simulink library "xbsEDKLib"  (Simulink 6.1)
libraries: xbsIndex_r4 x58
settings Model: LastModifiedBy=sps

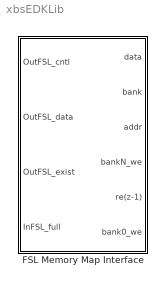
== system xbsEDKLib ==
  FSL Memory Map Interface : Subsystem
      settings: CopyFcn=set_param(gcbh,'LinkStatus','none');
      mask Display:
      | fprintf('','COMMENT: begin icon graphics {110:209:XBlock}');
      | patch([0 110 110 0 ],[0 0 209 209 ],[0.77 0.82 0.91]);
      | patch([25 7 33 7 25 54 62 70 101 76 53 36 61 36 53 76 101 70 62 54 25 ],[61 79 105 131 149 149 141 149 149 124 147 130 105 80 63 86 61 61 69 61 61 ],[.98 .96 .92]);
      | plot([0 0 110 110 0 ],[0 209 209 0 0 ]);
      | fprintf('','COMMENT: end icon graphics');
      | port_label('input',1,'OutFSL_cntl');
      | port_label('input',2,'OutFSL_data');
      | port_label('input',3,'OutFSL_exist');
      | port_label('input',4,'InFSL_full');
      | 
      | port_label('output',1,'data');
      | port_label('output',2,'bank');
      | port_label('output',3,'addr');
      | port_label('output',4,'bankN_we');
      | port_label('output',5,'re(z-1)');
      | port_label('output',6,'bank0_we');

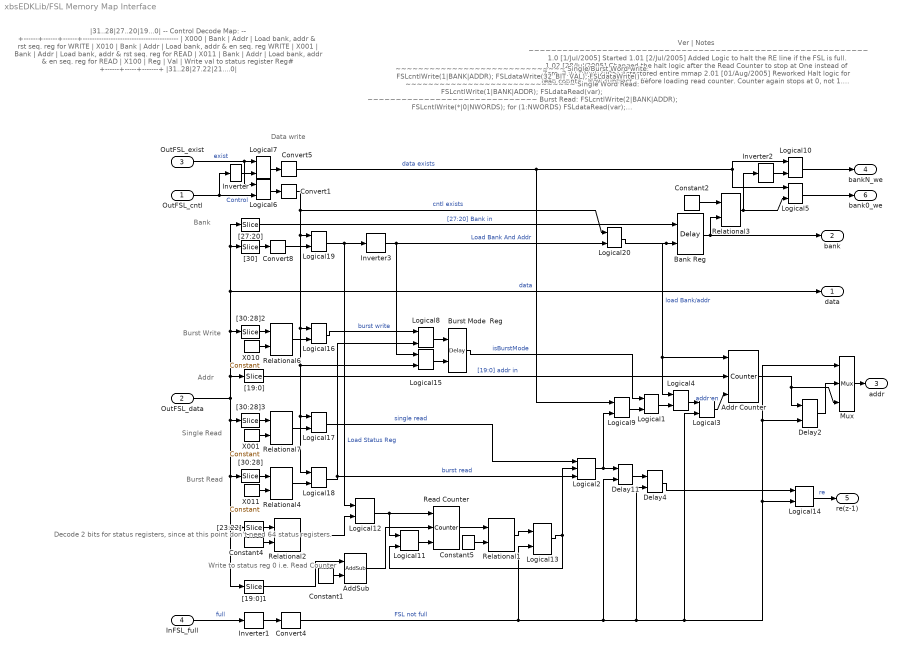
== system xbsEDKLib/FSL Memory Map Interface ==
  note: Ver | Notes
      | ~~~~~~~~~~~~~~~~~~~~~~~~~~~~~~~~~~~~~~~~~~~~~~~~~~~~~~~~~~~~
      | 1.0   [1/Jul/2005] Started
      | 1.01  [2/Jul/2005] Added Logic to halt the RE line if the FSL
      |       is full.
      | 1.02  [28/Jul/2005] Changed the halt logic after the Read
      |       Counter to stop at One instead of Zero.
      | 2.0   [30/Jul/2005] Refactored entire mmap
      | 2.01  [01/Aug/2005] Reworked Halt logic for read counter. Now
      |       subtract 1 before loading read counter. Counter again
      |       stops at 0, not 1. Subtract 1 from Read Count: since
      |       single/array read will cause one pulse.
      | 2.02  [18/Sep/2005] Added re(z-2) for FIFO reads
  note: ~~~~~~~~~~~~~~~~~~~~~~~~~~~~~~
      | Single/Burst Word write:
      |    FSLcntlWrite(1|BANK|ADDR);
      |    FSLdataWrite(32_BIT_VAL);
      |    FSLdataWrite() ...
      | ~~~~~~~~~~~~~~~~~~~~~~~~~~~~~~
      | Single Word Read:
      |    FSLcntlWrite(1|BANK|ADDR);
      |    FSLdataRead(var);
      | ~~~~~~~~~~~~~~~~~~~~~~~~~~~~~~
      | Burst Read:
      |    FSLcntlWrite(2|BANK|ADDR);
      |    FSLcntlWrite(*|0|NWORDS);
      |    for (1:NWORDS)
      |      FSLdataRead(var);
      | ~~~~~~~~~~~~~~~~~~~~~~~~~~~~~~
      | For RAM *=3, FIFO *=1
  note: |31..28|27..20|19...0|  -- Control Decode Map: --
      | +------+------+------+-----------------------------------------
      | | X000 | Bank | Addr | Load bank, addr & rst seq. reg for WRITE
      | | X010 | Bank | Addr | Load bank, addr & en seq. reg WRITE
      | | X001 | Bank | Addr | Load bank, addr & rst seq. reg for READ
      | | X011 | Bank | Addr | Load bank, addr & en seq. reg for READ
      | | X100 | Reg |  Val  | Write val to status register Reg#
      | +------+-----+-------+
      | |31..28|27.22|21....0|
  note: Write to status reg 0
      | i.e. Read Counter
  note: Burst
      | Read
  note: Decode 2 bits for
      | status registers,
      | since at this point
      | don't need 64
      |  status registers.
  note: Data write
  note: Burst
      | Write
  note: Single
      | Read
  note: Bank
  note: Addr
  OutFSL_cntl : Inport  Port=1  LatchInput=off
  OutFSL_data : Inport  Port=2  LatchInput=off
  OutFSL_exist : Inport  Port=3  LatchInput=off
  InFSL_full : Inport  Port=4  LatchInput=off
  AddSub : xbsIndex_r4/AddSub  mode=Subtraction  use_carryin=off  use_carryout=off  en=off  latency=0  precision=User Defined  arith_type=Unsigned  n_bits=20  bin_pt=0  quantization=Truncate  overflow=Wrap  dbl_ovrd=off  use_behavioral_HDL=off  pipelined=off  use_rpm=on  block_type=addsub
      settings: block_version=VER_STRING_GOES_HERE
  Addr Counter : xbsIndex_r4/Counter  cnt_type=Free Running  cnt_to=Inf  operation=Up  start_count=0  cnt_by_val=1  arith_type=Unsigned  n_bits=20  bin_pt=0  load_pin=on  rst=off  en=on  dbl_ovrd=off  explicit_period=off  period=1  use_behavioral_HDL=off  use_rpm=off  block_type=counter
      settings: infoedit="Configurable up, down and up/down counter.<P><P>Hardware notes: Free running counters are the least expensive in hardware.  A count limited counter is implemented by combining a counter with a comparator."  block_version=VER_STRING_GOES_HERE
  Bank Reg : xbsIndex_r4/Delay  en=on  latency=1  dbl_ovrd=off  reg_retiming=on  block_type=delay
      settings: infoedit="Delay line having  configurable length.<P><P>Hardware notes: A delay line is a chain, each link of which is an SRL16 followed by a flip-flop. If register retiming is enabled, the delay line is a chain of flip-flops."  block_version=VER_STRING_GOES_HERE
  Burst Mode  Reg : xbsIndex_r4/Delay  en=on  latency=1  dbl_ovrd=off  reg_retiming=on  block_type=delay
      settings: infoedit="Delay line having  configurable length.<P><P>Hardware notes: A delay line is a chain, each link of which is an SRL16 followed by a flip-flop. If register retiming is enabled, the delay line is a chain of flip-flops."  block_version=VER_STRING_GOES_HERE
  Constant1 : xbsIndex_r4/Constant  arith_type=Unsigned  const=1  n_bits=8  bin_pt=0  explicit_period=off  period=1  equ=P=C  opselect=C  inp2=PCIN>>17  opr=+  inp1=P  carry=CIN  dbl_ovrd=off  block_type=constant
      settings: block_version=VER_STRING_GOES_HERE
  Constant2 : xbsIndex_r4/Constant  arith_type=Unsigned  const=0  n_bits=8  bin_pt=0  explicit_period=off  period=1  equ=P=C  opselect=C  inp2=PCIN>>17  opr=+  inp1=P  carry=CIN  dbl_ovrd=off  block_type=constant
      settings: block_version=VER_STRING_GOES_HERE
  Constant4 : xbsIndex_r4/Constant  arith_type=Unsigned  const=0  n_bits=2  bin_pt=0  explicit_period=off  period=1  equ=P=C  opselect=C  inp2=PCIN>>17  opr=+  inp1=P  carry=CIN  dbl_ovrd=off  block_type=constant
      settings: block_version=VER_STRING_GOES_HERE
  Constant5 : xbsIndex_r4/Constant  arith_type=Unsigned  const=0  n_bits=20  bin_pt=0  explicit_period=off  period=1  equ=P=C  opselect=C  inp2=PCIN>>17  opr=+  inp1=P  carry=CIN  dbl_ovrd=off  block_type=constant
      settings: block_version=VER_STRING_GOES_HERE
  Convert{1,4..5,8} (4 alike) : xbsIndex_r4/Convert  arith_type=Boolean  n_bits=8  bin_pt=6  quantization=Truncate  overflow=Wrap  latency=0  dbl_ovrd=off  pipeline=off  block_type=convert
      settings: infoedit=The input is presented at the output after quantization and overflow effects.<P><P>Hardware notes: Additional hardware is used when rounding or saturation is selected and output width is less than the input width.  block_version=VER_STRING_GOES_HERE
  Delay11 : xbsIndex_r4/Delay  en=on  latency=1  dbl_ovrd=off  reg_retiming=on  block_type=delay
      settings: infoedit="Delay line having  configurable length.<P><P>Hardware notes: A delay line is a chain, each link of which is an SRL16 followed by a flip-flop. If register retiming is enabled, the delay line is a chain of flip-flops."  block_version=VER_STRING_GOES_HERE
  Delay2 : xbsIndex_r4/Delay  en=on  latency=1  dbl_ovrd=off  reg_retiming=on  block_type=delay
      settings: infoedit="Delay line having  configurable length.<P><P>Hardware notes: A delay line is a chain, each link of which is an SRL16 followed by a flip-flop. If register retiming is enabled, the delay line is a chain of flip-flops."  block_version=VER_STRING_GOES_HERE
  Delay4 : xbsIndex_r4/Delay  en=on  latency=1  dbl_ovrd=off  reg_retiming=on  block_type=delay
      settings: infoedit="Delay line having  configurable length.<P><P>Hardware notes: A delay line is a chain, each link of which is an SRL16 followed by a flip-flop. If register retiming is enabled, the delay line is a chain of flip-flops."  block_version=VER_STRING_GOES_HERE
  Inverter{,1..3} (4 alike) : xbsIndex_r4/Inverter  en=off  latency=0  dbl_ovrd=off  block_type=inv
      settings: block_version=VER_STRING_GOES_HERE
  Logical{1,3,15..20} (8 alike) : xbsIndex_r4/Logical  logical_function=AND  inputs=2  en=off  latency=0  precision=Full  arith_type=Unsigned  n_bits=1  bin_pt=0  align_bp=off  dbl_ovrd=off  block_type=logical
      settings: block_version=VER_STRING_GOES_HERE
  Logical{5,10,12..14} (5 alike) : xbsIndex_r4/Logical  logical_function=AND  inputs=2  en=off  latency=0  precision=Full  arith_type=Unsigned  n_bits=8  bin_pt=2  align_bp=on  dbl_ovrd=off  block_type=logical
      settings: block_version=VER_STRING_GOES_HERE
  Logical11 : xbsIndex_r4/Logical  logical_function=OR  inputs=2  en=off  latency=0  precision=Full  arith_type=Unsigned  n_bits=8  bin_pt=2  align_bp=on  dbl_ovrd=off  block_type=logical
      settings: block_version=VER_STRING_GOES_HERE
  Logical2 : xbsIndex_r4/Logical  logical_function=OR  inputs=3  en=off  latency=0  precision=Full  arith_type=Unsigned  n_bits=8  bin_pt=2  align_bp=on  dbl_ovrd=off  block_type=logical
      settings: block_version=VER_STRING_GOES_HERE
  Logical4 : xbsIndex_r4/Logical  logical_function=OR  inputs=2  en=off  latency=0  precision=Full  arith_type=Unsigned  n_bits=1  bin_pt=0  align_bp=off  dbl_ovrd=off  block_type=logical
      settings: block_version=VER_STRING_GOES_HERE
  Logical6 : xbsIndex_r4/Logical  logical_function=AND  inputs=2  en=off  latency=0  precision=User Defined  arith_type=Unsigned  n_bits=1  bin_pt=0  align_bp=off  dbl_ovrd=off  block_type=logical
      settings: block_version=VER_STRING_GOES_HERE
  Logical7 : xbsIndex_r4/Logical  logical_function=AND  inputs=2  en=off  latency=0  precision=User Defined  arith_type=Unsigned  n_bits=1  bin_pt=0  align_bp=off  dbl_ovrd=off  block_type=logical
      settings: block_version=VER_STRING_GOES_HERE
  Logical8 : xbsIndex_r4/Logical  logical_function=OR  inputs=2  en=off  latency=0  precision=Full  arith_type=Unsigned  n_bits=8  bin_pt=2  align_bp=on  dbl_ovrd=off  block_type=logical
      settings: block_version=VER_STRING_GOES_HERE
  Logical9 : xbsIndex_r4/Logical  logical_function=OR  inputs=2  en=off  latency=0  precision=Full  arith_type=Unsigned  n_bits=1  bin_pt=0  align_bp=off  dbl_ovrd=off  block_type=logical
      settings: block_version=VER_STRING_GOES_HERE
  Mux : xbsIndex_r4/Mux  inputs=2  en=off  latency=0  precision=Full  arith_type=Unsigned  n_bits=8  bin_pt=2  quantization=Truncate  overflow=Wrap  dbl_ovrd=off  block_type=mux
      settings: block_version=VER_STRING_GOES_HERE
  Read Counter : xbsIndex_r4/Counter  cnt_type=Free Running  cnt_to=Inf  operation=Down  start_count=0  cnt_by_val=1  arith_type=Unsigned  n_bits=20  bin_pt=0  load_pin=on  rst=off  en=on  dbl_ovrd=off  explicit_period=off  period=1  use_behavioral_HDL=off  use_rpm=off  block_type=counter
      settings: infoedit="Configurable up, down and up/down counter.<P><P>Hardware notes: Free running counters are the least expensive in hardware.  A count limited counter is implemented by combining a counter with a comparator."  block_version=VER_STRING_GOES_HERE
  Relational1 : xbsIndex_r4/Relational  mode=a!=b  en=off  latency=0  dbl_ovrd=off  block_type=relational
      settings: block_version=VER_STRING_GOES_HERE
  Relational{2..4,6..7} (5 alike) : xbsIndex_r4/Relational  mode=a=b  en=off  latency=0  dbl_ovrd=off  block_type=relational
      settings: block_version=VER_STRING_GOES_HERE
  X001 : xbsIndex_r4/Constant  arith_type=Unsigned  const=1  n_bits=3  bin_pt=0  explicit_period=off  period=1  equ=P=C  opselect=C  inp2=PCIN>>17  opr=+  inp1=P  carry=CIN  dbl_ovrd=off  block_type=constant
      settings: block_version=VER_STRING_GOES_HERE
  X010 : xbsIndex_r4/Constant  arith_type=Unsigned  const=2  n_bits=3  bin_pt=0  explicit_period=off  period=1  equ=P=C  opselect=C  inp2=PCIN>>17  opr=+  inp1=P  carry=CIN  dbl_ovrd=off  block_type=constant
      settings: block_version=VER_STRING_GOES_HERE
  X011 : xbsIndex_r4/Constant  arith_type=Unsigned  const=3  n_bits=3  bin_pt=0  explicit_period=off  period=1  equ=P=C  opselect=C  inp2=PCIN>>17  opr=+  inp1=P  carry=CIN  dbl_ovrd=off  block_type=constant
      settings: block_version=VER_STRING_GOES_HERE
  "[19:0]" : xbsIndex_r4/Slice  nbits=20  boolean_output=off  mode=Lower Bit Location + Width  bit1=19  base1=LSB of Input  bit0=0  base0=LSB of Input  dbl_ovrd=off  block_type=slice
      settings: infoedit="Extracts a given range of bits from each input sample and presents it at the output.  The output type is ordinarily unsigned with binary point at zero, but can be Boolean when the slice is one bit wide.<P><P>Hardware notes: In hardware this block costs nothing."  block_version=VER_STRING_GOES_HERE
  "[19:0]1" : xbsIndex_r4/Slice  nbits=24  boolean_output=off  mode=Two Bit Locations  bit1=19  base1=LSB of Input  bit0=0  base0=LSB of Input  dbl_ovrd=off  block_type=slice
      settings: infoedit="Extracts a given range of bits from each input sample and presents it at the output.  The output type is ordinarily unsigned with binary point at zero, but can be Boolean when the slice is one bit wide.<P><P>Hardware notes: In hardware this block costs nothing."  block_version=VER_STRING_GOES_HERE
  "[23:22]" : xbsIndex_r4/Slice  nbits=24  boolean_output=off  mode=Two Bit Locations  bit1=23  base1=LSB of Input  bit0=22  base0=LSB of Input  dbl_ovrd=off  block_type=slice
      settings: infoedit="Extracts a given range of bits from each input sample and presents it at the output.  The output type is ordinarily unsigned with binary point at zero, but can be Boolean when the slice is one bit wide.<P><P>Hardware notes: In hardware this block costs nothing."  block_version=VER_STRING_GOES_HERE
  "[27:20]" : xbsIndex_r4/Slice  nbits=8  boolean_output=off  mode=Lower Bit Location + Width  bit1=19  base1=LSB of Input  bit0=20  base0=LSB of Input  dbl_ovrd=off  block_type=slice
      settings: infoedit="Extracts a given range of bits from each input sample and presents it at the output.  The output type is ordinarily unsigned with binary point at zero, but can be Boolean when the slice is one bit wide.<P><P>Hardware notes: In hardware this block costs nothing."  block_version=VER_STRING_GOES_HERE
  "[30:28]" : xbsIndex_r4/Slice  nbits=3  boolean_output=off  mode=Lower Bit Location + Width  bit1=19  base1=LSB of Input  bit0=28  base0=LSB of Input  dbl_ovrd=off  block_type=slice
      settings: infoedit="Extracts a given range of bits from each input sample and presents it at the output.  The output type is ordinarily unsigned with binary point at zero, but can be Boolean when the slice is one bit wide.<P><P>Hardware notes: In hardware this block costs nothing."  block_version=VER_STRING_GOES_HERE
  "[30:28]2" : xbsIndex_r4/Slice  nbits=3  boolean_output=off  mode=Lower Bit Location + Width  bit1=19  base1=LSB of Input  bit0=28  base0=LSB of Input  dbl_ovrd=off  block_type=slice
      settings: infoedit="Extracts a given range of bits from each input sample and presents it at the output.  The output type is ordinarily unsigned with binary point at zero, but can be Boolean when the slice is one bit wide.<P><P>Hardware notes: In hardware this block costs nothing."  block_version=VER_STRING_GOES_HERE
  "[30:28]3" : xbsIndex_r4/Slice  nbits=3  boolean_output=off  mode=Lower Bit Location + Width  bit1=19  base1=LSB of Input  bit0=28  base0=LSB of Input  dbl_ovrd=off  block_type=slice
      settings: infoedit="Extracts a given range of bits from each input sample and presents it at the output.  The output type is ordinarily unsigned with binary point at zero, but can be Boolean when the slice is one bit wide.<P><P>Hardware notes: In hardware this block costs nothing."  block_version=VER_STRING_GOES_HERE
  "[30]" : xbsIndex_r4/Slice  nbits=1  boolean_output=off  mode=Lower Bit Location + Width  bit1=19  base1=LSB of Input  bit0=30  base0=LSB of Input  dbl_ovrd=off  block_type=slice
      settings: infoedit="Extracts a given range of bits from each input sample and presents it at the output.  The output type is ordinarily unsigned with binary point at zero, but can be Boolean when the slice is one bit wide.<P><P>Hardware notes: In hardware this block costs nothing."  block_version=VER_STRING_GOES_HERE
  data : Outport
  bank : Outport  Port=2
  addr : Outport  Port=3
  bankN_we : Outport  Port=4
  re(z-1) : Outport  Port=5
  bank0_we : Outport  Port=6
  wires:
  Logical2/1 -> Delay11/1, Logical9/2
  Logical5/1 -> bank0_we/1
  Relational3/1 -> Logical5/2, Inverter2/1
  Constant2/1 -> Relational3/1
  Delay11/1 -> Delay4/1
  Convert1/1 -> Logical19/1, Logical16/1, Logical17/1, Logical18/1, Logical15/2, Logical20/1  "cntl exists"
  X011/1 -> Relational4/2
  "[30:28]"/1 -> Relational4/1
  Addr Counter/1 -> Delay2/1, Mux/3
  Bank Reg/1 -> Relational3/2, bank/1
  Convert4/1 -> Delay11/2, Delay4/2, Logical3/2, Logical14/2, Delay2/2, Mux/1, Logical13/2  "FSL not full"
  InFSL_full/1 -> Inverter1/1  "full"
  Inverter1/1 -> Convert4/1
  Logical13/1 -> Logical2/2, Logical11/2
  Logical11/1 -> Read Counter/3
  Constant5/1 -> Relational1/2
  Read Counter/1 -> Relational1/1
  Logical12/1 -> Logical11/1, Read Counter/1
  "[23:22]"/1 -> Relational2/1
  Constant4/1 -> Relational2/2
  OutFSL_data/1 -> "[30:28]"/1, "[23:22]"/1, "[19:0]1"/1, "[30:28]3"/1, "[19:0]"/1, "[30:28]2"/1, "[27:20]"/1, "[30]"/1, data/1  "data"
  Convert5/1 -> Logical9/1, Logical5/1, Logical10/1  "data exists"
  OutFSL_cntl/1 -> Logical6/2, Inverter/1  "Control"
  Inverter/1 -> Logical7/2
  Logical6/1 -> Convert1/1
  Logical7/1 -> Convert5/1
  Relational2/1 -> Logical12/2
  Logical14/1 -> re(z-1)/1  "re"
  X010/1 -> Relational6/2
  "[30:28]2"/1 -> Relational6/1
  Relational6/1 -> Logical16/2
  X001/1 -> Relational7/2
  "[30:28]3"/1 -> Relational7/1
  Relational7/1 -> Logical17/2
  OutFSL_exist/1 -> Logical7/1, Logical6/1  "exist"
  Relational4/1 -> Logical18/2
  "[30]"/1 -> Convert8/1
  Logical19/1 -> Inverter3/1, Logical12/1  "Load Status Reg"
  Inverter3/1 -> Logical15/1, Logical20/2  "Load Bank And Addr"
  "[27:20]"/1 -> Bank Reg/1  "[27:20] Bank in"
  "[19:0]"/1 -> Addr Counter/2  "[19:0] addr in"
  Logical1/1 -> Logical4/2
  Logical8/1 -> Burst Mode  Reg/1
  Logical16/1 -> Logical8/1  "burst write"
  Logical18/1 -> Logical8/2, Logical2/3  "burst read"
  Burst Mode  Reg/1 -> Logical1/1  "isBurstMode"
  Logical9/1 -> Logical1/2
  Logical17/1 -> Logical2/1  "single read"
  Logical4/1 -> Logical3/1
  Logical3/1 -> Addr Counter/3  "addr en"
  Inverter2/1 -> Logical10/2
  Logical10/1 -> bankN_we/1
  Convert8/1 -> Logical19/2
  Delay4/1 -> Logical14/1
  Logical15/1 -> Burst Mode  Reg/2
  Logical20/1 -> Bank Reg/2, Logical4/1, Addr Counter/1  "load Bank/addr"
  AddSub/1 -> Read Counter/2
  Constant1/1 -> AddSub/2
  "[19:0]1"/1 -> AddSub/1
  Mux/1 -> addr/1
  Delay2/1 -> Mux/2
  Relational1/1 -> Logical13/1
